simulink library "dhp"  (Simulink 8.2)
settings: Solver=ode45  SolverMode=SingleTasking  StartTime=0.0  StopTime=10.0  RelTol=1e-3
undefined symbols (not defined in the file or in its folder): KDHP_DisableOBDAnnoun_flg, KDHP_SystemFaultHOTimer_sec, KDHP_SystemFaultRPTimer_sec
settings Model: Creator=13192  LastModifiedBy=14014

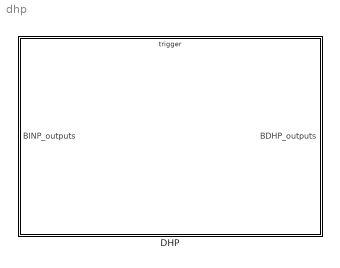
== system dhp ==
  DHP : Subsystem
      settings: RTWSystemCode=Nonreusable function  RTWFcnNameOpts=Use subsystem name  RTWFileNameOpts=Use subsystem name

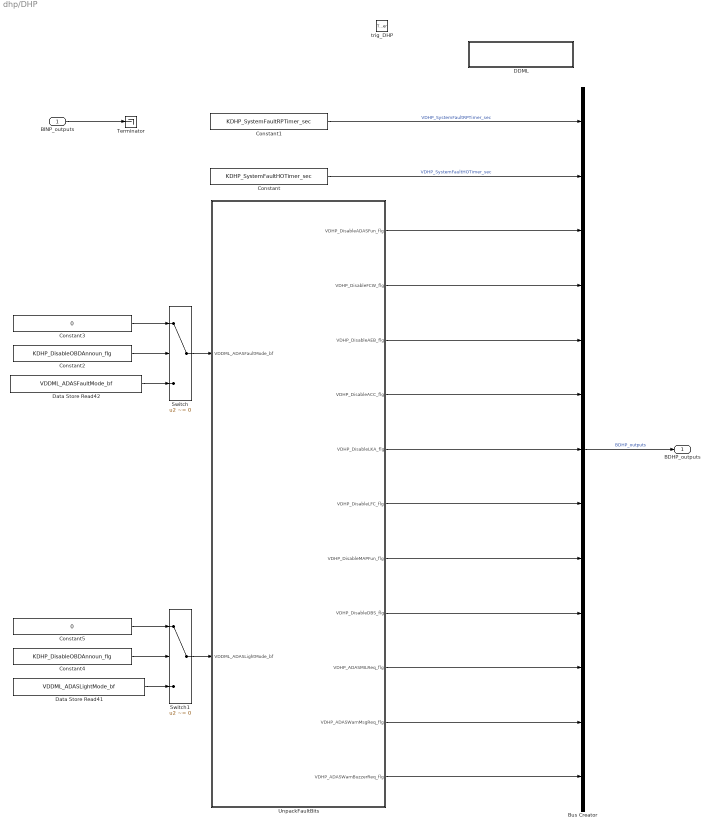
== system dhp/DHP ==
  BINP_outputs : Inport  OutDataTypeStr=Bus: BINP_outputs
  trig_DHP : TriggerPort  TriggerType=function-call
  Bus Creator : BusCreator  Inputs=13  OutDataTypeStr=Bus: BDHP_outputs
  Constant : Constant  Value=KDHP_SystemFaultHOTimer_sec
  Constant1 : Constant  Value=KDHP_SystemFaultRPTimer_sec
  Constant2 : Constant  Value=KDHP_DisableOBDAnnoun_flg
  Constant3 : Constant  Value=0  OutDataTypeStr=uint16
  Constant4 : Constant  Value=KDHP_DisableOBDAnnoun_flg
  Constant5 : Constant  Value=0  OutDataTypeStr=uint16
  DDML : Subsystem
      mask Display: disp('DDML Parameters')
  Data Store Read41 : DataStoreRead  DataStoreName=VDDML_ADASLightMode_bf
  Data Store Read42 : DataStoreRead  DataStoreName=VDDML_ADASFaultMode_bf
  Switch : Switch  Criteria=u2 ~= 0
  Switch1 : Switch  Criteria=u2 ~= 0
  Terminator : Terminator
  UnpackFaultBits : Subsystem
  BDHP_outputs : Outport  OutDataTypeStr=Bus: BDHP_outputs
  wires:
  Bus Creator/1 -> BDHP_outputs/1  "BDHP_outputs"
  Constant/1 -> Bus Creator/2  "VDHP_SystemFaultHOTimer_sec"
  Data Store Read42/1 -> Switch/3
  Data Store Read41/1 -> Switch1/3
  UnpackFaultBits/1(VDHP_DisableADASFun_flg) -> Bus Creator/3
  UnpackFaultBits/3(VDHP_DisableAEB_flg) -> Bus Creator/5
  UnpackFaultBits/4(VDHP_DisableACC_flg) -> Bus Creator/6
  UnpackFaultBits/6(VDHP_DisableLFC_flg) -> Bus Creator/8
  UnpackFaultBits/2(VDHP_DisableFCW_flg) -> Bus Creator/4
  UnpackFaultBits/5(VDHP_DisableLKA_flg) -> Bus Creator/7
  UnpackFaultBits/7(VDHP_DisableMAPFun_flg) -> Bus Creator/9
  UnpackFaultBits/9(VDHP_ADASMILReq_flg) -> Bus Creator/11
  BINP_outputs/1 -> Terminator/1
  UnpackFaultBits/11(VDHP_ADASWarnBuzzerReq_flg) -> Bus Creator/13
  Constant1/1 -> Bus Creator/1  "VDHP_SystemFaultRPTimer_sec"
  Switch/1 -> UnpackFaultBits/1(VDDML_ADASFaultMode_bf)
  Constant2/1 -> Switch/2
  Constant3/1 -> Switch/1
  Constant4/1 -> Switch1/2
  Constant5/1 -> Switch1/1
  Switch1/1 -> UnpackFaultBits/2(VDDML_ADASLightMode_bf)
  UnpackFaultBits/10(VDHP_ADASWarnMsgReq_flg) -> Bus Creator/12
  UnpackFaultBits/8(VDHP_DisableDBS_flg) -> Bus Creator/10

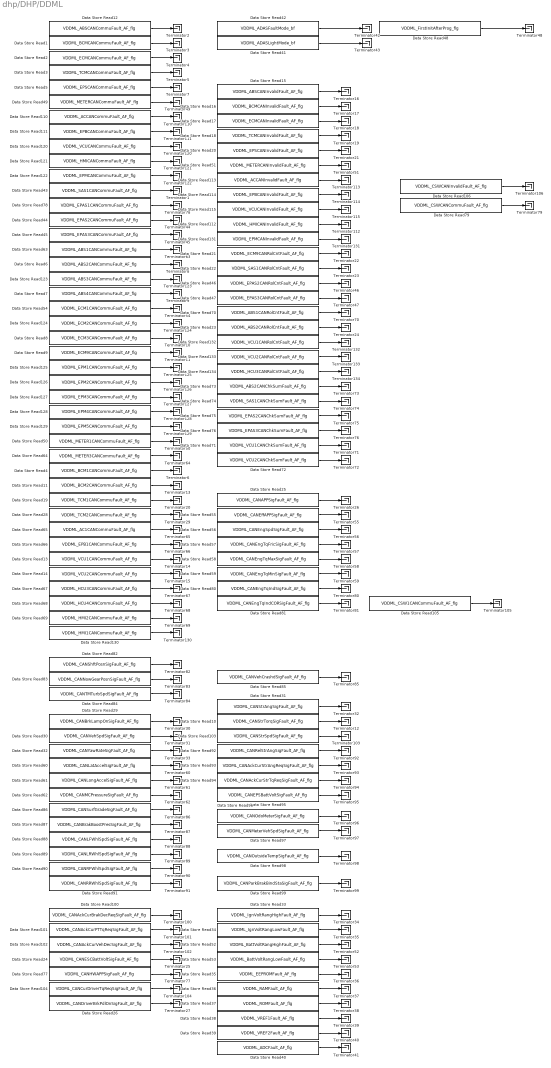
== system dhp/DHP/DDML ==
  Data Store Read1 : DataStoreRead  DataStoreName=VDDML_BCMCANCommuFault_AF_flg
  Data Store Read10 : DataStoreRead  DataStoreName=VDDML_CANStrTorqSigFault_AF_flg
  Data Store Read100 : DataStoreRead  DataStoreName=VDDML_CANAckCurBrakDecReqSigFault_AF_flg
  Data Store Read101 : DataStoreRead  DataStoreName=VDDML_CANAckCurPTTqReqSigFault_AF_flg
  Data Store Read102 : DataStoreRead  DataStoreName=VDDML_CANAckCurVehDecSigFault_AF_flg
  Data Store Read103 : DataStoreRead  DataStoreName=VDDML_CANStrSpdSigFault_AF_flg
  Data Store Read104 : DataStoreRead  DataStoreName=VDDML_CANCurDriverTqReqSigFault_AF_flg
  Data Store Read105 : DataStoreRead  DataStoreName=VDDML_CSW1CANCommuFault_AF_flg
  Data Store Read106 : DataStoreRead  DataStoreName=VDDML_CSWCANInvalidFault_AF_flg
  Data Store Read11 : DataStoreRead  DataStoreName=VDDML_BCM2CANCommuFault_AF_flg
  Data Store Read110 : DataStoreRead  DataStoreName=VDDML_ACCANCommuFault_AF_flg
  Data Store Read111 : DataStoreRead  DataStoreName=VDDML_EPBCANCommuFault_AF_flg
  Data Store Read112 : DataStoreRead  DataStoreName=VDDML_HMICANInvalidFault_AF_flg
  Data Store Read113 : DataStoreRead  DataStoreName=VDDML_ACCANInvalidFault_AF_flg
  Data Store Read114 : DataStoreRead  DataStoreName=VDDML_EPBCANInvalidFault_AF_flg
  Data Store Read115 : DataStoreRead  DataStoreName=VDDML_VCUCANInvalidFault_AF_flg
  Data Store Read12 : DataStoreRead  DataStoreName=VDDML_ABSCANCommuFault_AF_flg
  Data Store Read120 : DataStoreRead  DataStoreName=VDDML_VCUCANCommuFault_AF_flg
  Data Store Read121 : DataStoreRead  DataStoreName=VDDML_HMICANCommuFault_AF_flg
  Data Store Read122 : DataStoreRead  DataStoreName=VDDML_EPMCANCommuFault_AF_flg
  Data Store Read123 : DataStoreRead  DataStoreName=VDDML_ABS3CANCommuFault_AF_flg
  Data Store Read124 : DataStoreRead  DataStoreName=VDDML_ECM2CANCommuFault_AF_flg
  Data Store Read125 : DataStoreRead  DataStoreName=VDDML_EPM1CANCommuFault_AF_flg
  Data Store Read126 : DataStoreRead  DataStoreName=VDDML_EPM2CANCommuFault_AF_flg
  Data Store Read127 : DataStoreRead  DataStoreName=VDDML_EPM3CANCommuFault_AF_flg
  Data Store Read128 : DataStoreRead  DataStoreName=VDDML_EPM4CANCommuFault_AF_flg
  Data Store Read129 : DataStoreRead  DataStoreName=VDDML_EPM5CANCommuFault_AF_flg
  Data Store Read13 : DataStoreRead  DataStoreName=VDDML_VCU1CANCommuFault_AF_flg
  Data Store Read130 : DataStoreRead  DataStoreName=VDDML_HMI1CANCommuFault_AF_flg
  Data Store Read131 : DataStoreRead  DataStoreName=VDDML_EPMCANInvalidFault_AF_flg
  Data Store Read132 : DataStoreRead  DataStoreName=VDDML_VCU1CANRolCntFault_AF_flg
  Data Store Read133 : DataStoreRead  DataStoreName=VDDML_VCU2CANRolCntFault_AF_flg
  Data Store Read134 : DataStoreRead  DataStoreName=VDDML_HCU3CANRolCntFault_AF_flg
  Data Store Read14 : DataStoreRead  DataStoreName=VDDML_VCU2CANCommuFault_AF_flg
  Data Store Read15 : DataStoreRead  DataStoreName=VDDML_ABSCANInvalidFault_AF_flg
  Data Store Read16 : DataStoreRead  DataStoreName=VDDML_BCMCANInvalidFault_AF_flg
  Data Store Read17 : DataStoreRead  DataStoreName=VDDML_ECMCANInvalidFault_AF_flg
  Data Store Read18 : DataStoreRead  DataStoreName=VDDML_TCMCANInvalidFault_AF_flg
  Data Store Read19 : DataStoreRead  DataStoreName=VDDML_TCM1CANCommuFault_AF_flg
  Data Store Read2 : DataStoreRead  DataStoreName=VDDML_ECMCANCommuFault_AF_flg
  Data Store Read20 : DataStoreRead  DataStoreName=VDDML_EPSCANInvalidFault_AF_flg
  Data Store Read21 : DataStoreRead  DataStoreName=VDDML_ECM9CANRolCntFault_AF_flg
  Data Store Read22 : DataStoreRead  DataStoreName=VDDML_SAS1CANRolCntFault_AF_flg
  Data Store Read23 : DataStoreRead  DataStoreName=VDDML_ABS2CANRolCntFault_AF_flg
  Data Store Read24 : DataStoreRead  DataStoreName=VDDML_CANESCBattVoltSigFault_AF_flg
  Data Store Read25 : DataStoreRead  DataStoreName=VDDML_CANAPPSigFault_AF_flg
  Data Store Read26 : DataStoreRead  DataStoreName=VDDML_CANDriverBrkPdlOnSigFault_AF_flg
  Data Store Read28 : DataStoreRead  DataStoreName=VDDML_TCM2CANCommuFault_AF_flg
  Data Store Read29 : DataStoreRead  DataStoreName=VDDML_CANBrkLampOnSigFault_AF_flg
  Data Store Read3 : DataStoreRead  DataStoreName=VDDML_TCMCANCommuFault_AF_flg
  Data Store Read30 : DataStoreRead  DataStoreName=VDDML_CANVehSpdSigFault_AF_flg
  Data Store Read31 : DataStoreRead  DataStoreName=VDDML_CANStrAngSigFault_AF_flg
  Data Store Read32 : DataStoreRead  DataStoreName=VDDML_CANYawRateSigFault_AF_flg
  Data Store Read33 : DataStoreRead  DataStoreName=VDDML_IgnVoltRangHighFault_AF_flg
  Data Store Read34 : DataStoreRead  DataStoreName=VDDML_IgnVoltRangLowFault_AF_flg
  Data Store Read35 : DataStoreRead  DataStoreName=VDDML_EEPROMFault_AF_flg
  Data Store Read36 : DataStoreRead  DataStoreName=VDDML_RAMFault_AF_flg
  Data Store Read37 : DataStoreRead  DataStoreName=VDDML_ROMFault_AF_flg
  Data Store Read38 : DataStoreRead  DataStoreName=VDDML_VREF1Fault_AF_flg
  Data Store Read39 : DataStoreRead  DataStoreName=VDDML_VREF2Fault_AF_flg
  Data Store Read4 : DataStoreRead  DataStoreName=VDDML_BCM1CANCommuFault_AF_flg
  Data Store Read40 : DataStoreRead  DataStoreName=VDDML_ADCFault_AF_flg
  Data Store Read41 : DataStoreRead  DataStoreName=VDDML_ADASLightMode_bf
  Data Store Read42 : DataStoreRead  DataStoreName=VDDML_ADASFaultMode_bf
  Data Store Read43 : DataStoreRead  DataStoreName=VDDML_SAS1CANCommuFault_AF_flg
  Data Store Read44 : DataStoreRead  DataStoreName=VDDML_EPAS2CANCommuFault_AF_flg
  Data Store Read45 : DataStoreRead  DataStoreName=VDDML_EPAS3CANCommuFault_AF_flg
  Data Store Read46 : DataStoreRead  DataStoreName=VDDML_EPAS2CANRolCntFault_AF_flg
  Data Store Read47 : DataStoreRead  DataStoreName=VDDML_EPAS3CANRolCntFault_AF_flg
  Data Store Read48 : DataStoreRead  DataStoreName=VDDML_FirstInitAfterProg_flg
  Data Store Read49 : DataStoreRead  DataStoreName=VDDML_METERCANCommuFault_AF_flg
  Data Store Read5 : DataStoreRead  DataStoreName=VDDML_EPSCANCommuFault_AF_flg
  Data Store Read50 : DataStoreRead  DataStoreName=VDDML_METER1CANCommuFault_AF_flg
  Data Store Read51 : DataStoreRead  DataStoreName=VDDML_METERCANInvalidFault_AF_flg
  Data Store Read52 : DataStoreRead  DataStoreName=VDDML_BattVoltRangHighFault_AF_flg
  Data Store Read53 : DataStoreRead  DataStoreName=VDDML_BattVoltRangLowFault_AF_flg
  Data Store Read54 : DataStoreRead  DataStoreName=VDDML_ECM1CANCommuFault_AF_flg
  Data Store Read55 : DataStoreRead  DataStoreName=VDDML_CANEffAPPSigFault_AF_flg
  Data Store Read56 : DataStoreRead  DataStoreName=VDDML_CANEngSpdSigFault_AF_flg
  Data Store Read57 : DataStoreRead  DataStoreName=VDDML_CANEngTqFricSigFault_AF_flg
  Data Store Read58 : DataStoreRead  DataStoreName=VDDML_CANEngTqMaxSigFault_AF_flg
  Data Store Read59 : DataStoreRead  DataStoreName=VDDML_CANEngTqMinSigFault_AF_flg
  Data Store Read6 : DataStoreRead  DataStoreName=VDDML_ABS2CANCommuFault_AF_flg
  Data Store Read60 : DataStoreRead  DataStoreName=VDDML_CANLatAccelSigFault_AF_flg
  Data Store Read61 : DataStoreRead  DataStoreName=VDDML_CANLongAccelSigFault_AF_flg
  Data Store Read62 : DataStoreRead  DataStoreName=VDDML_CANMCPressureSigFault_AF_flg
  Data Store Read63 : DataStoreRead  DataStoreName=VDDML_ABS1CANCommuFault_AF_flg
  Data Store Read64 : DataStoreRead  DataStoreName=VDDML_METER3CANCommuFault_AF_flg
  Data Store Read65 : DataStoreRead  DataStoreName=VDDML_AC1CANCommuFault_AF_flg
  Data Store Read66 : DataStoreRead  DataStoreName=VDDML_EPB1CANCommuFault_AF_flg
  Data Store Read67 : DataStoreRead  DataStoreName=VDDML_HCU3CANCommuFault_AF_flg
  Data Store Read68 : DataStoreRead  DataStoreName=VDDML_HCU4CANCommuFault_AF_flg
  Data Store Read69 : DataStoreRead  DataStoreName=VDDML_HMI2CANCommuFault_AF_flg
  Data Store Read7 : DataStoreRead  DataStoreName=VDDML_ABS4CANCommuFault_AF_flg
  Data Store Read70 : DataStoreRead  DataStoreName=VDDML_ABS1CANRolCntFault_AF_flg
  Data Store Read71 : DataStoreRead  DataStoreName=VDDML_VCU1CANChkSumFault_AF_flg
  Data Store Read72 : DataStoreRead  DataStoreName=VDDML_VCU2CANChkSumFault_AF_flg
  Data Store Read73 : DataStoreRead  DataStoreName=VDDML_ABS2CANChkSumFault_AF_flg
  Data Store Read74 : DataStoreRead  DataStoreName=VDDML_SAS1CANChkSumFault_AF_flg
  Data Store Read75 : DataStoreRead  DataStoreName=VDDML_EPAS2CANChkSumFault_AF_flg
  Data Store Read76 : DataStoreRead  DataStoreName=VDDML_EPAS3CANChkSumFault_AF_flg
  Data Store Read77 : DataStoreRead  DataStoreName=VDDML_CANHWAPPSigFault_AF_flg
  Data Store Read78 : DataStoreRead  DataStoreName=VDDML_EPAS1CANCommuFault_AF_flg
  Data Store Read79 : DataStoreRead  DataStoreName=VDDML_CSWCANCommuFault_AF_flg
  Data Store Read8 : DataStoreRead  DataStoreName=VDDML_ECM3CANCommuFault_AF_flg
  Data Store Read80 : DataStoreRead  DataStoreName=VDDML_CANEngTqIndSigFault_AF_flg
  Data Store Read81 : DataStoreRead  DataStoreName=VDDML_CANEngTqIndCORSigFault_AF_flg
  Data Store Read82 : DataStoreRead  DataStoreName=VDDML_CANShftPosnSigFault_AF_flg
  Data Store Read83 : DataStoreRead  DataStoreName=VDDML_CANNowGearPosnSigFault_AF_flg
  Data Store Read84 : DataStoreRead  DataStoreName=VDDML_CANTMTurbSpdSigFault_AF_flg
  Data Store Read85 : DataStoreRead  DataStoreName=VDDML_CANVehCrashdSigFault_AF_flg
  Data Store Read86 : DataStoreRead  DataStoreName=VDDML_CANSurfGradeSigFault_AF_flg
  Data Store Read87 : DataStoreRead  DataStoreName=VDDML_CANBrakBoostPresSigFault_AF_flg
  Data Store Read88 : DataStoreRead  DataStoreName=VDDML_CANLFWhlSpdSigFault_AF_flg
  Data Store Read89 : DataStoreRead  DataStoreName=VDDML_CANLRWhlSpdSigFault_AF_flg
  Data Store Read9 : DataStoreRead  DataStoreName=VDDML_ECM9CANCommuFault_AF_flg
  Data Store Read90 : DataStoreRead  DataStoreName=VDDML_CANRFWhlSpdSigFault_AF_flg
  Data Store Read91 : DataStoreRead  DataStoreName=VDDML_CANRRWhlSpdSigFault_AF_flg
  Data Store Read92 : DataStoreRead  DataStoreName=VDDML_CANRelStrAngSigFault_AF_flg
  Data Store Read93 : DataStoreRead  DataStoreName=VDDML_CANAckCurStrAngReqSigFault_AF_flg
  Data Store Read94 : DataStoreRead  DataStoreName=VDDML_CANAckCurStrTqReqSigFault_AF_flg
  Data Store Read95 : DataStoreRead  DataStoreName=VDDML_CANEPSBattVoltSigFault_AF_flg
  Data Store Read96 : DataStoreRead  DataStoreName=VDDML_CANOdoMeterSigFault_AF_flg
  Data Store Read97 : DataStoreRead  DataStoreName=VDDML_CANMeterVehSpdSigFault_AF_flg
  Data Store Read98 : DataStoreRead  DataStoreName=VDDML_CANOutsideTempSigFault_AF_flg
  Data Store Read99 : DataStoreRead  DataStoreName=VDDML_CANParkBrakBindStaSigFault_AF_flg
  Terminator{1..27,29..106,110..115,120..134} (126 alike) : Terminator
  wires:
  Data Store Read12/1 -> Terminator2/1
  Data Store Read1/1 -> Terminator3/1
  Data Store Read2/1 -> Terminator4/1
  Data Store Read3/1 -> Terminator5/1
  Data Store Read6/1 -> Terminator8/1
  Data Store Read7/1 -> Terminator9/1
  Data Store Read8/1 -> Terminator10/1
  Data Store Read9/1 -> Terminator11/1
  Data Store Read15/1 -> Terminator16/1
  Data Store Read16/1 -> Terminator17/1
  Data Store Read17/1 -> Terminator18/1
  Data Store Read18/1 -> Terminator19/1
  Data Store Read20/1 -> Terminator21/1
  Data Store Read21/1 -> Terminator22/1
  Data Store Read22/1 -> Terminator23/1
  Data Store Read23/1 -> Terminator24/1
  Data Store Read25/1 -> Terminator26/1
  Data Store Read29/1 -> Terminator30/1
  Data Store Read30/1 -> Terminator31/1
  Data Store Read31/1 -> Terminator32/1
  Data Store Read32/1 -> Terminator33/1
  Data Store Read33/1 -> Terminator34/1
  Data Store Read34/1 -> Terminator35/1
  Data Store Read35/1 -> Terminator36/1
  Data Store Read36/1 -> Terminator37/1
  Data Store Read37/1 -> Terminator38/1
  Data Store Read38/1 -> Terminator39/1
  Data Store Read39/1 -> Terminator40/1
  Data Store Read40/1 -> Terminator41/1
  Data Store Read43/1 -> Terminator1/1
  Data Store Read5/1 -> Terminator7/1
  Data Store Read44/1 -> Terminator44/1
  Data Store Read45/1 -> Terminator45/1
  Data Store Read46/1 -> Terminator46/1
  Data Store Read47/1 -> Terminator47/1
  Data Store Read49/1 -> Terminator49/1
  Data Store Read50/1 -> Terminator50/1
  Data Store Read51/1 -> Terminator51/1
  Data Store Read52/1 -> Terminator52/1
  Data Store Read53/1 -> Terminator53/1
  Data Store Read54/1 -> Terminator54/1
  Data Store Read55/1 -> Terminator55/1
  Data Store Read56/1 -> Terminator56/1
  Data Store Read57/1 -> Terminator57/1
  Data Store Read58/1 -> Terminator58/1
  Data Store Read59/1 -> Terminator59/1
  Data Store Read60/1 -> Terminator60/1
  Data Store Read61/1 -> Terminator61/1
  Data Store Read62/1 -> Terminator62/1
  Data Store Read63/1 -> Terminator63/1
  Data Store Read10/1 -> Terminator12/1
  Data Store Read4/1 -> Terminator6/1
  Data Store Read11/1 -> Terminator13/1
  Data Store Read19/1 -> Terminator20/1
  Data Store Read28/1 -> Terminator29/1
  Data Store Read64/1 -> Terminator64/1
  Data Store Read65/1 -> Terminator65/1
  Data Store Read66/1 -> Terminator66/1
  Data Store Read70/1 -> Terminator70/1
  Data Store Read73/1 -> Terminator73/1
  Data Store Read74/1 -> Terminator74/1
  Data Store Read75/1 -> Terminator75/1
  Data Store Read76/1 -> Terminator76/1
  Data Store Read80/1 -> Terminator80/1
  Data Store Read81/1 -> Terminator81/1
  Data Store Read82/1 -> Terminator82/1
  Data Store Read83/1 -> Terminator83/1
  Data Store Read84/1 -> Terminator84/1
  Data Store Read85/1 -> Terminator85/1
  Data Store Read86/1 -> Terminator86/1
  Data Store Read87/1 -> Terminator87/1
  Data Store Read88/1 -> Terminator88/1
  Data Store Read89/1 -> Terminator89/1
  Data Store Read90/1 -> Terminator90/1
  Data Store Read91/1 -> Terminator91/1
  Data Store Read92/1 -> Terminator92/1
  Data Store Read93/1 -> Terminator93/1
  Data Store Read94/1 -> Terminator94/1
  Data Store Read95/1 -> Terminator95/1
  Data Store Read96/1 -> Terminator96/1
  Data Store Read97/1 -> Terminator97/1
  Data Store Read98/1 -> Terminator98/1
  Data Store Read99/1 -> Terminator99/1
  Data Store Read100/1 -> Terminator100/1
  Data Store Read101/1 -> Terminator101/1
  Data Store Read102/1 -> Terminator102/1
  Data Store Read110/1 -> Terminator110/1
  Data Store Read111/1 -> Terminator111/1
  Data Store Read113/1 -> Terminator113/1
  Data Store Read114/1 -> Terminator114/1
  Data Store Read115/1 -> Terminator115/1
  Data Store Read42/1 -> Terminator42/1
  Data Store Read41/1 -> Terminator43/1
  Data Store Read48/1 -> Terminator48/1
  Data Store Read120/1 -> Terminator120/1
  Data Store Read121/1 -> Terminator121/1
  Data Store Read122/1 -> Terminator122/1
  Data Store Read123/1 -> Terminator123/1
  Data Store Read124/1 -> Terminator124/1
  Data Store Read125/1 -> Terminator125/1
  Data Store Read126/1 -> Terminator126/1
  Data Store Read127/1 -> Terminator127/1
  Data Store Read128/1 -> Terminator128/1
  Data Store Read129/1 -> Terminator129/1
  Data Store Read13/1 -> Terminator14/1
  Data Store Read14/1 -> Terminator15/1
  Data Store Read67/1 -> Terminator67/1
  Data Store Read68/1 -> Terminator68/1
  Data Store Read69/1 -> Terminator69/1
  Data Store Read130/1 -> Terminator130/1
  Data Store Read112/1 -> Terminator112/1
  Data Store Read131/1 -> Terminator131/1
  Data Store Read132/1 -> Terminator132/1
  Data Store Read133/1 -> Terminator133/1
  Data Store Read134/1 -> Terminator134/1
  Data Store Read71/1 -> Terminator71/1
  Data Store Read72/1 -> Terminator72/1
  Data Store Read24/1 -> Terminator25/1
  Data Store Read77/1 -> Terminator77/1
  Data Store Read78/1 -> Terminator78/1
  Data Store Read103/1 -> Terminator103/1
  Data Store Read104/1 -> Terminator104/1
  Data Store Read105/1 -> Terminator105/1
  Data Store Read79/1 -> Terminator79/1
  Data Store Read106/1 -> Terminator106/1
  Data Store Read26/1 -> Terminator27/1

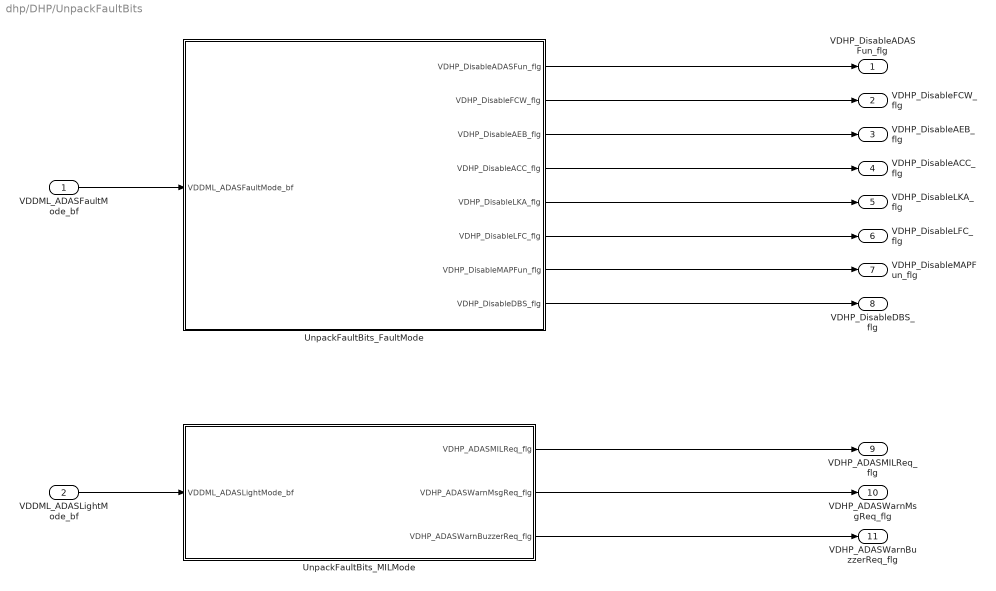
== system dhp/DHP/UnpackFaultBits ==
  VDDML_ADASFaultMode_bf : Inport
  VDDML_ADASLightMode_bf : Inport  Port=2
  UnpackFaultBits_FaultMode : Stateflow chart  TreatAsAtomicUnit=on
  UnpackFaultBits_MILMode : Stateflow chart  TreatAsAtomicUnit=on
  VDHP_DisableADASFun_flg : Outport
  VDHP_DisableFCW_flg : Outport  Port=2
  VDHP_DisableAEB_flg : Outport  Port=3
  VDHP_DisableACC_flg : Outport  Port=4
  VDHP_DisableLKA_flg : Outport  Port=5
  VDHP_DisableLFC_flg : Outport  Port=6
  VDHP_DisableMAPFun_flg : Outport  Port=7
  VDHP_DisableDBS_flg : Outport  Port=8
  VDHP_ADASMILReq_flg : Outport  Port=9
  VDHP_ADASWarnMsgReq_flg : Outport  Port=10
  VDHP_ADASWarnBuzzerReq_flg : Outport  Port=11
  wires:
  VDDML_ADASLightMode_bf/1 -> UnpackFaultBits_MILMode/1(VDDML_ADASLightMode_bf)
  UnpackFaultBits_FaultMode/4(VDHP_DisableACC_flg) -> VDHP_DisableACC_flg/1
  UnpackFaultBits_FaultMode/3(VDHP_DisableAEB_flg) -> VDHP_DisableAEB_flg/1
  UnpackFaultBits_FaultMode/1(VDHP_DisableADASFun_flg) -> VDHP_DisableADASFun_flg/1
  VDDML_ADASFaultMode_bf/1 -> UnpackFaultBits_FaultMode/1(VDDML_ADASFaultMode_bf)
  UnpackFaultBits_FaultMode/2(VDHP_DisableFCW_flg) -> VDHP_DisableFCW_flg/1
  UnpackFaultBits_FaultMode/5(VDHP_DisableLKA_flg) -> VDHP_DisableLKA_flg/1
  UnpackFaultBits_FaultMode/7(VDHP_DisableMAPFun_flg) -> VDHP_DisableMAPFun_flg/1
  UnpackFaultBits_MILMode/2(VDHP_ADASWarnMsgReq_flg) -> VDHP_ADASWarnMsgReq_flg/1
  UnpackFaultBits_MILMode/3(VDHP_ADASWarnBuzzerReq_flg) -> VDHP_ADASWarnBuzzerReq_flg/1
  UnpackFaultBits_MILMode/1(VDHP_ADASMILReq_flg) -> VDHP_ADASMILReq_flg/1
  UnpackFaultBits_FaultMode/6(VDHP_DisableLFC_flg) -> VDHP_DisableLFC_flg/1
  UnpackFaultBits_FaultMode/8(VDHP_DisableDBS_flg) -> VDHP_DisableDBS_flg/1

== stateflow chart DHP/UnpackFaultBits/UnpackFaultBits_MILMode ==
  (default) -> (junction 8) : {VDHP_ADASLightMode_bf =VDDML_ADASLightMode_bf ;}
  (junction 8) -> (junction 9) : {
      |     VDHP_ADASMILReq_flg                     = (VDHP_ADASLightMode_bf & 0x01) ;
      |     VDHP_ADASWarnMsgReq_flg           = (VDHP_ADASLightMode_bf & 0x04) >> 2;
      |     VDHP_ADASWarnBuzzerReq_flg      = (VDHP_ADASLightMode_bf & 0x10) >> 4;
      | }
  data: VDHP_ADASMILReq_flg output boolean; VDHP_ADASLightMode_bf local uint16; VDDML_ADASLightMode_bf input double; VDHP_ADASWarnMsgReq_flg output double; VDHP_ADASWarnBuzzerReq_flg output double
  data VDHP_ADASMILReq_flg settings: description=$TL$ name=$D; type=Bool; class=PROD_DISP; variable=DHP/VARS/VDHP_DisableStopStart_flg; $TL$
  data VDHP_ADASLightMode_bf settings: description=$TL$ name=$D; type=UInt16; class=PROD_DISP; variable=DHP/VARS/VDHP_HEVFaultMode_bf; scaling=VOID_SCALING; $TL$

== stateflow chart DHP/UnpackFaultBits/UnpackFaultBits_FaultMode ==
  note: Note:
      | 0 disable ADAS function
      | 1 disable FCW
      | 2 disable AEB
      | 3 disable ACC
      | 4 disable LKA
      | 5 disable LFC
      | 6 disable MAP function
      | 7 disable DBS
  (default) -> (junction 25) : {VDHP_ADASFaultMode_bf =VDDML_ADASFaultMode_bf ;}
  (junction 25) -> (junction 26) : {
      |     VDHP_DisableADASFun_flg         = (VDHP_ADASFaultMode_bf & 0x01) ;
      |     VDHP_DisableFCW_flg                 = (VDHP_ADASFaultMode_bf & 0x02) >> 1;
      |     VDHP_DisableAEB_flg                  = (VDHP_ADASFaultMode_bf & 0x04) >> 2;
      |     VDHP_DisableACC_flg                  = (VDHP_ADASFaultMode_bf & 0x08) >> 3 ;
      |     VDHP_DisableLKA_flg                  = (VDHP_ADASFaultMode_bf & 0x10) >> 4;
      |     VDHP_DisableLFC_flg                   = (VDHP_ADASFaultMode_bf & 0x20) >> 5;
      |     VDHP_DisableMAPFun_flg            = (VDHP_ADASFaultMode_bf & 0x40) >> 6;
      |     VDHP_DisableDBS_flg                  = (VDHP_ADASFaultMode_bf & 0x80) >> 7;
      | }
  data: VDHP_DisableADASFun_flg output boolean; VDHP_DisableFCW_flg output boolean; VDHP_DisableAEB_flg output boolean; VDHP_DisableACC_flg output boolean; VDHP_DisableLKA_flg output boolean; VDHP_DisableLFC_flg output boolean; VDHP_DisableMAPFun_flg output boolean; VDHP_ADASFaultMode_bf local uint16; VDDML_ADASFaultMode_bf input double; VDHP_DisableDBS_flg output double
  data VDHP_DisableADASFun_flg settings: description=$TL$ name=$D; type=Bool; class=PROD_DISP; variable=DHP/VARS/VDHP_DisableStopStart_flg; $TL$
  data VDHP_DisableFCW_flg settings: description=$TL$ name=$D; type=Bool; class=PROD_DISP; variable=DHP/VARS/VDHP_DisableHEV_flg; $TL$
  data VDHP_DisableAEB_flg settings: description=$TL$ name=$D; type=Bool; class=PROD_DISP; variable=DHP/VARS/VDHP_DisableRegen_flg; $TL$
  data VDHP_DisableACC_flg settings: description=$TL$ name=$D; type=Bool; class=PROD_DISP; variable=DHP/VARS/VDHP_DisableSmartCharge_flg; $TL$
  data VDHP_DisableLKA_flg settings: description=$TL$ name=$D; type=Bool; class=PROD_DISP; variable=DHP/VARS/VDHP_ForceLimpHome_flg; $TL$
  data VDHP_DisableLFC_flg settings: description=$TL$ name=$D; type=Bool; class=PROD_DISP; variable=DHP/VARS/VDHP_ForceConventional_flg; $TL$
  data VDHP_DisableMAPFun_flg settings: description=$TL$ name=$D; type=Bool; class=PROD_DISP; variable=DHP/VARS/VDHP_CriticalFault_flg; $TL$
  data VDHP_ADASFaultMode_bf settings: description=$TL$ name=$D; type=UInt16; class=PROD_DISP; variable=DHP/VARS/VDHP_HEVFaultMode_bf; scaling=VOID_SCALING; $TL$
